simulink model "derivative"  (R2017a)
settings: Solver=FixedStepDiscrete  StartTime=0.0  StopTime=Inf  RelTol=1e-3
undefined symbols (not defined in the file): none, videoinput
libraries: visionfilter x5, dspvision x1, imaqlib x1, visiontransforms x1
settings Model: SimulationMode=accelerator  Creator=eruffaldi  LastModifiedBy=eruffaldi
settings OptimizationCC: EfficientMapNaN2IntZero=off
settings HardwareCC: TargetBitPerLong=64  TargetBitPerPointer=64  TargetBitPerSizeT=64  TargetBitPerPtrDiffT=64  TargetLongLongMode=on  TargetIntDivRoundTo=Zero  TargetEndianess=LittleEndian  TargetWordSize=64  TargetHWDeviceType=MATLAB Host  ProdEqTarget=off
settings CodeAppCC: MaxIdLength=128
settings GRTTargetCC: TargetLangStandard=C89/C90 (ANSI)  CombineOutputUpdateFcns=off  GRTInterface=on

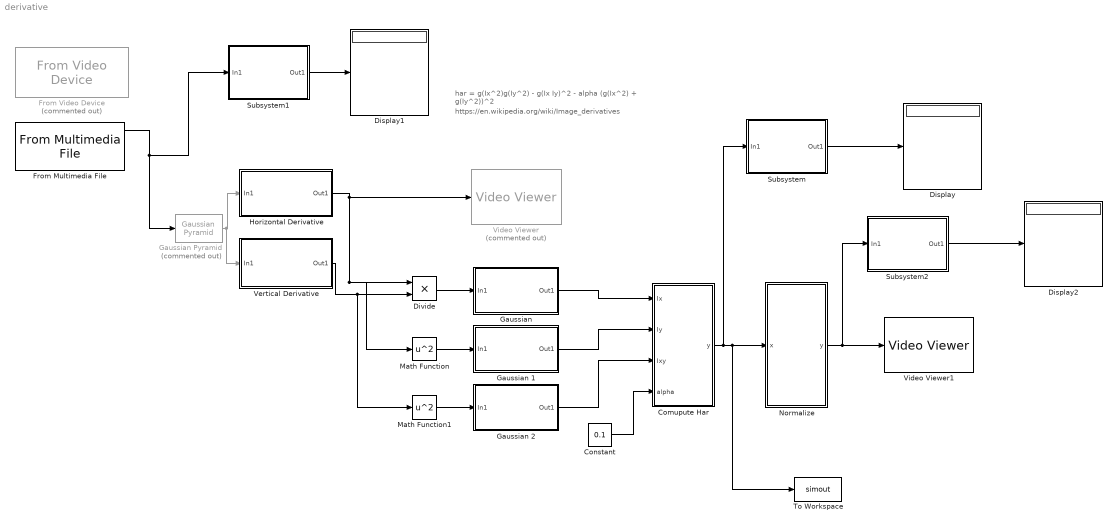
== system derivative ==
  note: har = g(Ix^2)g(Iy^2) - g(Ix Iy)^2 - alpha (g(Ix^2) + g(Iy^2))^2
  note: https://en.wikipedia.org/wiki/Image_derivatives
  Comupute Har : MATLAB Function  TreatAsAtomicUnit=on
  Constant : Constant  Value=0.1
  Display : Display
  Display1 : Display
  Display2 : Display
  Divide : Product  Inputs=**
  From Multimedia File : dspvision/From Multimedia File  inputFilename=/Users/eruffaldi/Dropbox/CourseSimulink/repo/examples/vision/SampleVideo_720x480_1mb.mp4  loop=on  numPlays=inf  outputStreams=Video only  videoDataType=single  audioDataType=int16  inheritSampleTime=on  userDefinedSampleTime=1/30  noAudioOutput=off  isIntensityVideo=off  fourcc=YCbCr 4:2:2  colorVideoFormat=One multidimensional signal  outputEOF=off  dataOrg=Column-major  audioFrameSize=1024  computeAudioFrameSize=off  outSamplingMode=Sample based
      settings: SourceProductBaseCode=VP
  From Video Device : imaqlib/From Video Device  Commented=on  DeviceMenu=macvideo 1 (FaceTime HD Camera)  Device=macvideo 1 (FaceTime HD Camera)  ObjConstructor=videoinput('macvideo', 1)  VideoFormatMenu=YCbCr422_1280x720  VideoFormat=YCbCr422_1280x720  VideoSource=default  ROIPosition=[0 0 720 1280]  EnableHWTrigger=off  TriggerConfiguration=none/none  SampleTime=1/30  OutputPortsMode=Separate color signals  DataType=single  CanDoHWTrigger=no  ReturnedColorSpace=YCbCr  BlockHandle=2235.0077  ROIWidth=1280  ROIHeight=720  ROIColumn=0  ROIRow=0  EngXMLPath=/Applications/MATLAB_R2017a.app/toolbox/imaq/imaq/private  DevXMLPath=/Users/eruffaldi/Documents/MATLAB/SupportPackages/R2017a/toolbox/imaq/supportpackages/genericvideo/adaptor/maci64  EngLibPath=/Applications/MATLAB_R2017a.app/toolbox/imaq/imaqblks/imaqmex/maci64  ColorSpace=YCbCr  BayerSensorAlignment=grbg
      settings: SourceProductName=Image Acquisition Toolbox
  "Gaussian " : Subsystem
  Gaussian 1 : Subsystem
  Gaussian 2 : Subsystem
  Gaussian Pyramid : visiontransforms/Gaussian Pyramid  Commented=on  operation=Reduce  level=1  source="Default separable filter [1/4-a/2  1/4  a  1/4  1/4-a/2]"  a=0.375  coef=[0.0625 0.25 0.375 0.25 0.0625]  hiddenCoef=[1/4-0.375/2 1/4 0.375 1/4 1/4-0.375/2]  firstCoeffMode=Specify word length  firstCoeffWordLength=16  firstCoeffFracLength=16  outputMode=Binary point scaling  outputWordLength=32  outputFracLength=10  prodOutputMode=Binary point scaling  prodOutputWordLength=32  prodOutputFracLength=10  roundingMode=Floor  overflowMode=off
      settings: SourceProductName=Computer Vision System Toolbox  SourceProductBaseCode=VP
  Horizontal Derivative : Subsystem
  Math Function : Math  Operator=square  SaturateOnIntegerOverflow=on
  Math Function1 : Math  Operator=square  SaturateOnIntegerOverflow=on
  Normalize : MATLAB Function  TreatAsAtomicUnit=on
  Subsystem : Subsystem
  Subsystem1 : Subsystem
  Subsystem2 : Subsystem
  To Workspace : ToWorkspace  VariableName=simout  SaveFormat=Timeseries  SampleTime=-1
      settings: MaxDataPoints=5
  Vertical Derivative : Subsystem
  Video Viewer : VideoViewer  Commented=on  FigPos=[280 769 846 595]
  Video Viewer1 : VideoViewer  FigPos=[1441 1074 1920 954]
  wires:
  Horizontal Derivative/1(Out1) -> Math Function/1, Divide/1, Video Viewer/1
  Vertical Derivative/1(Out1) -> Math Function1/1, Divide/2
  Divide/1 -> "Gaussian "/1(In1)
  Math Function/1 -> Gaussian 1/1(In1)
  Math Function1/1 -> Gaussian 2/1(In1)
  "Gaussian "/1(Out1) -> Comupute Har/1(Ix)
  Gaussian 1/1(Out1) -> Comupute Har/2(Iy)
  Gaussian 2/1(Out1) -> Comupute Har/3(Ixy)
  Constant/1 -> Comupute Har/4(alpha)
  Normalize/1(y) -> Subsystem2/1(In1), Video Viewer1/1
  Comupute Har/1(y) -> Subsystem/1(In1), To Workspace/1, Normalize/1(x)
  Gaussian Pyramid/1 -> Vertical Derivative/1(In1), Horizontal Derivative/1(In1)
  From Multimedia File/1 -> Subsystem1/1(In1), Gaussian Pyramid/1
  Subsystem/1(Out1) -> Display/1
  Subsystem1/1(Out1) -> Display1/1
  Subsystem2/1(Out1) -> Display2/1

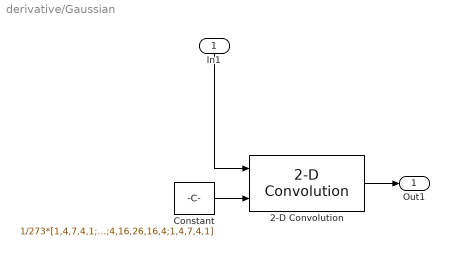
== system derivative/Gaussian  ==
  In1 : Inport
  2-D Convolution : visionfilter/2-D Convolution  outSize=Full  normalize=off  outputMode=Binary point scaling  outputWordLength=32  outputFracLength=12  prodOutputMode=Binary point scaling  prodOutputWordLength=32  prodOutputFracLength=10  roundingMode=Floor  overflowMode=off
      settings: SourceProductName=Computer Vision System Toolbox  SourceProductBaseCode=VP
  Constant : Constant  Value=1/273*[1,4,7,4,1;4,16,26,16,4;7,26,41,26,7;4,16,26,16,4;1,4,7,4,1]  OutDataTypeStr=single
  Out1 : Outport
  wires:
  In1/1 -> 2-D Convolution/1
  2-D Convolution/1 -> Out1/1
  Constant/1 -> 2-D Convolution/2

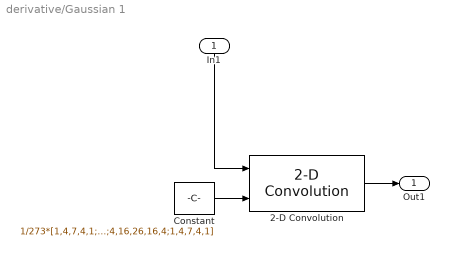
== system derivative/Gaussian 1 ==
  In1 : Inport
  2-D Convolution : visionfilter/2-D Convolution  outSize=Full  normalize=off  outputMode=Binary point scaling  outputWordLength=32  outputFracLength=12  prodOutputMode=Binary point scaling  prodOutputWordLength=32  prodOutputFracLength=10  roundingMode=Floor  overflowMode=off
      settings: SourceProductName=Computer Vision System Toolbox  SourceProductBaseCode=VP
  Constant : Constant  Value=1/273*[1,4,7,4,1;4,16,26,16,4;7,26,41,26,7;4,16,26,16,4;1,4,7,4,1]  OutDataTypeStr=single
  Out1 : Outport
  wires:
  In1/1 -> 2-D Convolution/1
  2-D Convolution/1 -> Out1/1
  Constant/1 -> 2-D Convolution/2

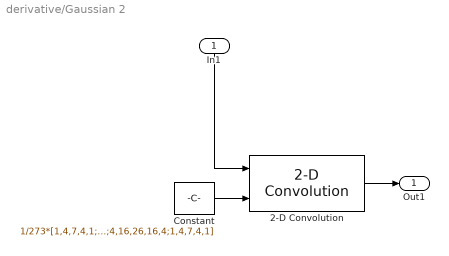
== system derivative/Gaussian 2 ==
  In1 : Inport
  2-D Convolution : visionfilter/2-D Convolution  outSize=Full  normalize=off  outputMode=Binary point scaling  outputWordLength=32  outputFracLength=12  prodOutputMode=Binary point scaling  prodOutputWordLength=32  prodOutputFracLength=10  roundingMode=Floor  overflowMode=off
      settings: SourceProductName=Computer Vision System Toolbox  SourceProductBaseCode=VP
  Constant : Constant  Value=1/273*[1,4,7,4,1;4,16,26,16,4;7,26,41,26,7;4,16,26,16,4;1,4,7,4,1]  OutDataTypeStr=single
  Out1 : Outport
  wires:
  In1/1 -> 2-D Convolution/1
  2-D Convolution/1 -> Out1/1
  Constant/1 -> 2-D Convolution/2

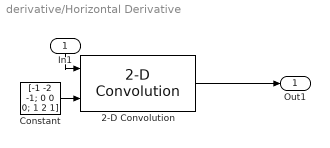
== system derivative/Horizontal Derivative ==
  In1 : Inport
  2-D Convolution : visionfilter/2-D Convolution  outSize=Full  normalize=off  outputMode=Binary point scaling  outputWordLength=32  outputFracLength=12  prodOutputMode=Binary point scaling  prodOutputWordLength=32  prodOutputFracLength=10  roundingMode=Floor  overflowMode=off
      settings: SourceProductName=Computer Vision System Toolbox  SourceProductBaseCode=VP
  Constant : Constant  Value=[-1 -2 -1; 0 0 0; 1 2 1]  OutDataTypeStr=single
  Out1 : Outport
  wires:
  2-D Convolution/1 -> Out1/1
  Constant/1 -> 2-D Convolution/2
  In1/1 -> 2-D Convolution/1

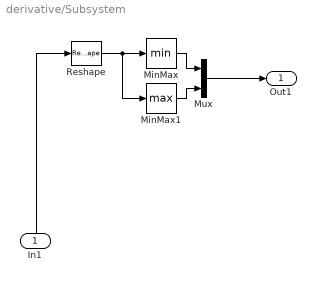
== system derivative/Subsystem ==
  In1 : Inport
  MinMax : MinMax
  MinMax1 : MinMax  Function=max
  Mux : Mux  Inputs=2
  Reshape : Reshape
  Out1 : Outport
  wires:
  MinMax1/1 -> Mux/2
  Reshape/1 -> MinMax1/1, MinMax/1
  Mux/1 -> Out1/1
  MinMax/1 -> Mux/1
  In1/1 -> Reshape/1

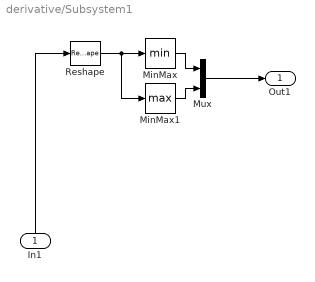
== system derivative/Subsystem1 ==
  In1 : Inport
  MinMax : MinMax
  MinMax1 : MinMax  Function=max
  Mux : Mux  Inputs=2
  Reshape : Reshape
  Out1 : Outport
  wires:
  MinMax1/1 -> Mux/2
  Reshape/1 -> MinMax1/1, MinMax/1
  Mux/1 -> Out1/1
  MinMax/1 -> Mux/1
  In1/1 -> Reshape/1

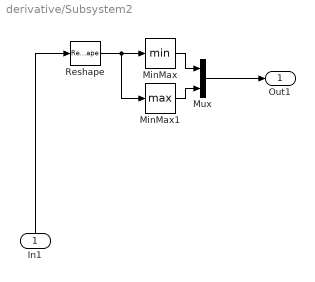
== system derivative/Subsystem2 ==
  In1 : Inport
  MinMax : MinMax
  MinMax1 : MinMax  Function=max
  Mux : Mux  Inputs=2
  Reshape : Reshape
  Out1 : Outport
  wires:
  MinMax1/1 -> Mux/2
  Reshape/1 -> MinMax1/1, MinMax/1
  Mux/1 -> Out1/1
  MinMax/1 -> Mux/1
  In1/1 -> Reshape/1

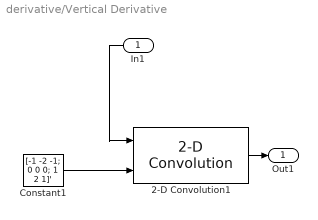
== system derivative/Vertical Derivative ==
  In1 : Inport
  2-D Convolution1 : visionfilter/2-D Convolution  outSize=Full  normalize=off  outputMode=Binary point scaling  outputWordLength=32  outputFracLength=12  prodOutputMode=Binary point scaling  prodOutputWordLength=32  prodOutputFracLength=10  roundingMode=Floor  overflowMode=off
      settings: SourceProductName=Computer Vision System Toolbox  SourceProductBaseCode=VP
  Constant1 : Constant  Value=[-1 -2 -1; 0 0 0; 1 2 1]'  OutDataTypeStr=single
  Out1 : Outport
  wires:
  Constant1/1 -> 2-D Convolution1/2
  In1/1 -> 2-D Convolution1/1
  2-D Convolution1/1 -> Out1/1

== matlab function derivative/Normalize ==
  data: x input; y output
function y = fcn(x)

w = log(abs(x));
f = w(:);
mi = min(f(f > -inf));
ma = max(f(f < inf));
y = (w-mi)/(ma-mi);

== matlab function derivative/Comupute Har ==
  data: Ix input; y output; Iy input; Ixy input; alpha input
function y = fcn(Ix,Iy,Ixy,alpha)

y = Ix.*Iy-Ixy.^2 - alpha * (Ix+Iy).^2;
